simulink model "tx_chain_test"  (R2022b)
settings: Solver=FixedStepDiscrete  StartTime=0.0  StopTime=inf  RelTol=1e-3
undefined symbols (not defined in the file or in its folder): S
libraries: simrfV2elements x7, simrfV2systems x2, rfTestbenches_lib x2
settings Model: Creator=hessam  LastModifiedBy=hessam
settings DebuggingCC: InheritedTsInSrcMsg=none

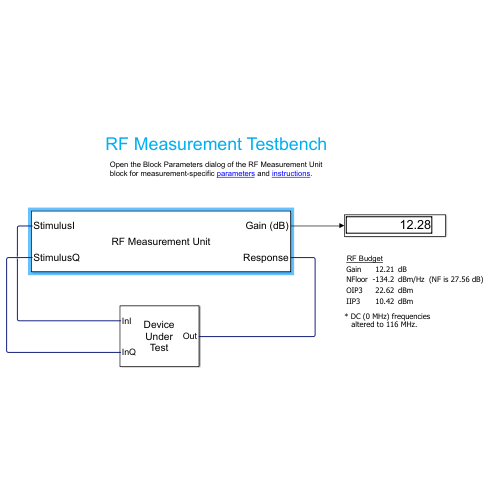
[thumbnail: Simulink's stored preview of the top-level diagram]
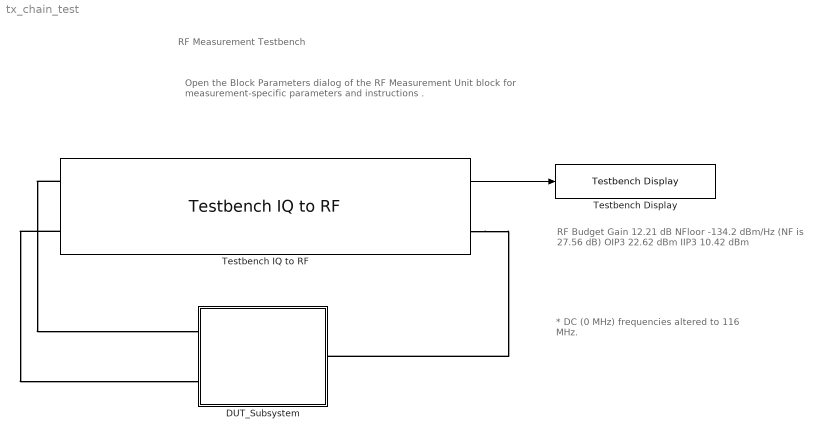
== system tx_chain_test ==
  note: RF Measurement Testbench
  note: Open the Block Parameters dialog of the RF Measurement Unit
      | block for measurement-specific parameters and instructions .
  note: * DC (0 MHz) frequencies
      | altered to 116 MHz.
  note: RF Budget
      |
      | Gain
      |
      | 12.21
      |
      | dB
      |
      | NFloor
      |
      | -134.2
      |
      | dBm/Hz
      |
      | (NF is 27.56 dB)
      |
      | OIP3
      |
      | 22.62
      |
      | dBm
      |
      | IIP3
      |
      | 10.42
      |
      | dBm
  DUT_Subsystem : Subsystem
      settings: LibrarySourceBlock=rfTestbenches_lib/simrfTestbenchIQtoRF/DUT_Subsystem
      mask Display: fprintf('Device\nUnder\nTest');
  Testbench Display : rfTestbenches_lib/simrfTestbenchIQtoRF/Testbench Display  Format=short
  Testbench IQ to RF : rfTestbenches_lib/Testbench IQ to RF  SimNoise=on  ModeStrLong=Gain  ModeStrShort=Sideband Suppression  Mode=1  IPTypeStr=Output referred  IPType=2  IQMeasureStr=I and Q (Q = -1j * I)  IQMeasure=1  InjectionTypeStr=Low-side  InjectionType=1  T_amp_dBm=0  T_amp_dBm_scL=-10  T_amp_dBm_scU=15  T_amp_dBmV=47  Fin=116e6  Fout=77e9  Base_bw=116e6  F_tone_over_Base_bw=1/8  Reset=0  ResetableRand=6.2788496288347118e-01
  wires:
  Testbench IQ to RF/1 -> Testbench Display/1
  connections:
  Testbench IQ to RF/RConn1 -- DUT_Subsystem/RConn1
  Testbench IQ to RF/LConn1 -- DUT_Subsystem/LConn1
  Testbench IQ to RF/LConn2 -- DUT_Subsystem/LConn2

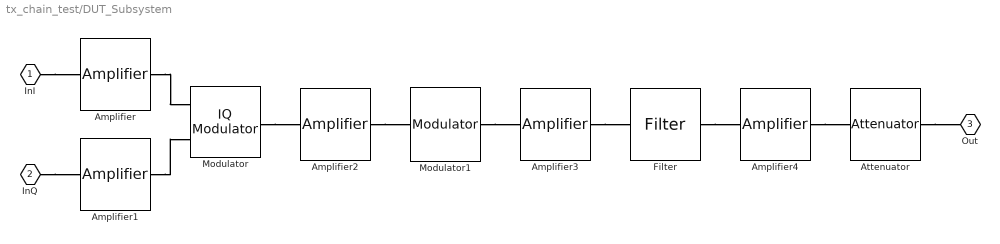
== system tx_chain_test/DUT_Subsystem ==
  Amplifier : simrfV2elements/Amplifier  classname=amplifier  DataSource=Data file  isNetworkObj=off  Paramtype=S-parameters  Sparam=[0 0;1 0]  SparamFreq=1e9 Hz  SparamZ0=50  isRationalObj=off  Residues=0  Poles=0  DF={0 0; 1 0}  Source_linear_gain=Available power gain  linear_gain=0 dB  AmAmAmPmTable=[-25,5,-1;-10,20,-2;0,27,5;5,28,12]  Zin=50  Zout=50  Source_Poly=Even and odd order  Poly_Coeffs=[0 1]  IPType=Output  IP2=Inf dBm  IP3=Inf dBm  P1dB=inf dBm  Psat=inf dBm  Gcomp=inf dBm  InternalGrounding=on  SourceFreq=Extracted from data source  PlotFreq=[1e9:1e6:3e9] Hz  PlotType=X-Y plane  YParam1=S(1,1)  YFormat1=Magnitude (dB)  YParam2=None  YFormat2=Magnitude (dB)  YOption=Linear  XOption=Linear  SparamRepresentation=Time domain (rationalfit)  FitTol=-40  FitOpt=Fit individually  MaxPoles=48  AutoImpulseLength=on  ImpulseLength=1e-10 s  MagModeling=off  AddNoise=on  NoiseType=Noise figure  NoiseDist=White  NF=25  MinNF=0  Gopt=0  RN=0  CarrierFreq=0 Hz  NoiseAutoImpulseLength=on  NoiseImpulseLength=1e-10 s  ConstS21NL=off  OpFreq=1 GHz  SetOpFreqAsMaxS21=off
  Amplifier1 : simrfV2elements/Amplifier  classname=amplifier  DataSource=Data file  isNetworkObj=off  Paramtype=S-parameters  Sparam=[0 0;1 0]  SparamFreq=1e9 Hz  SparamZ0=50  isRationalObj=off  Residues=0  Poles=0  DF={0 0; 1 0}  Source_linear_gain=Available power gain  linear_gain=0 dB  AmAmAmPmTable=[-25,5,-1;-10,20,-2;0,27,5;5,28,12]  Zin=50  Zout=50  Source_Poly=Even and odd order  Poly_Coeffs=[0 1]  IPType=Output  IP2=Inf dBm  IP3=Inf dBm  P1dB=inf dBm  Psat=inf dBm  Gcomp=inf dBm  InternalGrounding=on  SourceFreq=Extracted from data source  PlotFreq=[1e9:1e6:3e9] Hz  PlotType=X-Y plane  YParam1=S(1,1)  YFormat1=Magnitude (dB)  YParam2=None  YFormat2=Magnitude (dB)  YOption=Linear  XOption=Linear  SparamRepresentation=Time domain (rationalfit)  FitTol=-40  FitOpt=Fit individually  MaxPoles=48  AutoImpulseLength=on  ImpulseLength=1e-10 s  MagModeling=off  AddNoise=on  NoiseType=Noise figure  NoiseDist=White  NF=25  MinNF=0  Gopt=0  RN=0  CarrierFreq=0 Hz  NoiseAutoImpulseLength=on  NoiseImpulseLength=1e-10 s  ConstS21NL=off  OpFreq=1 GHz  SetOpFreqAsMaxS21=off
  Amplifier2 : simrfV2elements/Amplifier  classname=amplifier  DataSource=Data file  isNetworkObj=off  Paramtype=S-parameters  Sparam=[0 0;1 0]  SparamFreq=1e9 Hz  SparamZ0=50  isRationalObj=off  Residues=0  Poles=0  DF={0 0; 1 0}  Source_linear_gain=Available power gain  linear_gain=5 dB  AmAmAmPmTable=[-25,5,-1;-10,20,-2;0,27,5;5,28,12]  Zin=50  Zout=50  Source_Poly=Even and odd order  Poly_Coeffs=[0 1]  IPType=Output  IP2=Inf dBm  IP3=25 dBm  P1dB=inf dBm  Psat=inf dBm  Gcomp=inf dBm  InternalGrounding=on  SourceFreq=Extracted from data source  PlotFreq=[1e9:1e6:3e9] Hz  PlotType=X-Y plane  YParam1=S(1,1)  YFormat1=Magnitude (dB)  YParam2=None  YFormat2=Magnitude (dB)  YOption=Linear  XOption=Linear  SparamRepresentation=Time domain (rationalfit)  FitTol=-40  FitOpt=Fit individually  MaxPoles=48  AutoImpulseLength=on  ImpulseLength=1e-10 s  MagModeling=off  AddNoise=on  NoiseType=Noise figure  NoiseDist=White  NF=15  MinNF=0  Gopt=0  RN=0  CarrierFreq=0 Hz  NoiseAutoImpulseLength=on  NoiseImpulseLength=1e-10 s  ConstS21NL=off  OpFreq=1 GHz  SetOpFreqAsMaxS21=off
  Amplifier3 : simrfV2elements/Amplifier  classname=amplifier  DataSource=Data file  isNetworkObj=off  Paramtype=S-parameters  Sparam=[0 0;1 0]  SparamFreq=1e9 Hz  SparamZ0=50  isRationalObj=off  Residues=0  Poles=0  DF={0 0; 1 0}  Source_linear_gain=Available power gain  linear_gain=9 dB  AmAmAmPmTable=[-25,5,-1;-10,20,-2;0,27,5;5,28,12]  Zin=50  Zout=50  Source_Poly=Even and odd order  Poly_Coeffs=[0 1]  IPType=Output  IP2=Inf dBm  IP3=25 dBm  P1dB=inf dBm  Psat=inf dBm  Gcomp=inf dBm  InternalGrounding=on  SourceFreq=Extracted from data source  PlotFreq=[1e9:1e6:3e9] Hz  PlotType=X-Y plane  YParam1=S(1,1)  YFormat1=Magnitude (dB)  YParam2=None  YFormat2=Magnitude (dB)  YOption=Linear  XOption=Linear  SparamRepresentation=Time domain (rationalfit)  FitTol=-40  FitOpt=Fit individually  MaxPoles=48  AutoImpulseLength=on  ImpulseLength=1e-10 s  MagModeling=off  AddNoise=on  NoiseType=Noise figure  NoiseDist=White  NF=15  MinNF=0  Gopt=0  RN=0  CarrierFreq=0 Hz  NoiseAutoImpulseLength=on  NoiseImpulseLength=1e-10 s  ConstS21NL=off  OpFreq=1 GHz  SetOpFreqAsMaxS21=off
  Amplifier4 : simrfV2elements/Amplifier  classname=amplifier  DataSource=Data file  isNetworkObj=off  Paramtype=S-parameters  Sparam=[0 0;1 0]  SparamFreq=1e9 Hz  SparamZ0=50  isRationalObj=off  Residues=0  Poles=0  DF={0 0; 1 0}  Source_linear_gain=Available power gain  linear_gain=10 dB  AmAmAmPmTable=[-25,5,-1;-10,20,-2;0,27,5;5,28,12]  Zin=50  Zout=50  Source_Poly=Even and odd order  Poly_Coeffs=[0 1]  IPType=Output  IP2=Inf dBm  IP3=40 dBm  P1dB=inf dBm  Psat=inf dBm  Gcomp=inf dBm  InternalGrounding=on  SourceFreq=Extracted from data source  PlotFreq=[1e9:1e6:3e9] Hz  PlotType=X-Y plane  YParam1=S(1,1)  YFormat1=Magnitude (dB)  YParam2=None  YFormat2=Magnitude (dB)  YOption=Linear  XOption=Linear  SparamRepresentation=Time domain (rationalfit)  FitTol=-40  FitOpt=Fit individually  MaxPoles=48  AutoImpulseLength=on  ImpulseLength=1e-10 s  MagModeling=off  AddNoise=on  NoiseType=Noise figure  NoiseDist=White  NF=25  MinNF=0  Gopt=0  RN=0  CarrierFreq=0 Hz  NoiseAutoImpulseLength=on  NoiseImpulseLength=1e-10 s  ConstS21NL=off  OpFreq=1 GHz  SetOpFreqAsMaxS21=off
  Attenuator : simrfV2elements/Attenuator  classname=attenuator  Att=4  Zin=50  Zout=50  AddNoise=on  InternalGrounding=on
  Filter : simrfV2elements/Filter  classname=filter  DesignMethod=Butterworth  ResponseType=Bandstop  Implementation=LC Tee  ImplementationIdeal=Constant per carrier  ImplementationRational=Transfer function  UseFilterOrder=on  FilterOrder=3  PassFreq_lp=1 GHz  PassFreq_hp=2 GHz  PassFreq_bp=[2 3] GHz  PassFreq_bs=[1 4] GHz  PassAtten=10*log10(2)  StopFreq_lp=2 GHz  StopFreq_hp=1 GHz  StopFreq_bp=[1.5 3.5] GHz  StopFreq_bs=[51 55] GHz  StopAtten=40  Rsrc=100  Rload=50  AutoImpulseLength=on  ImpulseLength=1e-10 s  InternalGrounding=on  PlotFuncLeft=Voltage transfer  PlotLeftForm=Magnitude (dB)  PlotRightOnVT=None  PlotRightNoTD=None  PlotRightNoGD=None  PlotRightNoIR=None  PlotRightNoSR=None  PlotRightForm=Magnitude (dB)  FreqPoints=logspace(0,10,101)  Freq_unit=Hz  TimePoints=linspace(0,1,1e6+1)  Time_unit=s  XaxisScale=Linear  YaxisScale=Linear  needRedraw=0
  Modulator : simrfV2systems/IQ Modulator  classname=iqmod  Source_linear_gain=Available power gain  linear_gain=1 dB  Poly_Coeffs=[0 1]  LOFreq=10.884 GHz  Zin=50  Zout=50  AddIRFilters=on  AddCSFilter=on  InternalGrounding=on  ForceNextInit=off  NFloor=-149.865494556439  GainMismatch=0 dB  PhaseMismatch=0 deg  Isolation=inf dB  AddPhaseNoise=off  PhaseNoiseOffset=1  PhaseNoiseLevel=-Inf  AutoImpulseLengthPN=on  ImpulseLengthPN=1e-10  ImpulseLength_unitPN=s  Source_Poly=Even and odd order  IPType=Output  IP2=Inf dBm  IP3=15 dBm  P1dB=inf dBm  Psat=inf dBm  Gcomp=inf dBm  DesignMethodIR=Ideal  ResponseTypeIR=Lowpass  ImplementationIR=LC Tee  ImplementationIdealIR=Constant per carrier  ImplementationRationalIR=Transfer function  UseFilterOrderIR=on  FilterOrderIR=3  PassFreq_lpIR=174  PassFreq_lp_unitIR=MHz  PassFreq_hpIR=58  PassFreq_hp_unitIR=MHz  PassFreq_bpIR=[58 174]  PassFreq_bp_unitIR=MHz  PassFreq_bsIR=[21.825999999 21.942000001]  PassFreq_bs_unitIR=GHz  PassAttenIR=10*log10(2)  StopFreq_lpIR=174.000001  StopFreq_lp_unitIR=MHz  StopFreq_hpIR=57.999999  StopFreq_hp_unitIR=MHz  StopFreq_bpIR=[57.999999 174.000001]  StopFreq_bp_unitIR=MHz  StopFreq_bsIR=[21.826 21.942]  StopFreq_bs_unitIR=GHz  StopAttenIR=40  RsrcIR=50  RloadIR=50  AutoImpulseLengthIR=on  ImpulseLengthIR=1e-10  ImpulseLength_unitIR=s  DesignMethodCS=Ideal  ResponseTypeCS=Highpass  ImplementationCS=LC Tee  ImplementationIdealCS=Constant per carrier  ImplementationRationalCS=Transfer function  UseFilterOrderCS=on  FilterOrderCS=3  PassFreq_lpCS=11.058  PassFreq_lp_unitCS=GHz  PassFreq_hpCS=10.942  PassFreq_hp_unitCS=GHz  PassFreq_bpCS=[10.942 11.058]  PassFreq_bp_unitCS=GHz  PassFreq_bsCS=[10.709999999 10.826000001]  PassFreq_bs_unitCS=GHz  PassAttenCS=10*log10(2)  StopFreq_lpCS=11.058000001  StopFreq_lp_unitCS=GHz  StopFreq_hpCS=10.941999999  StopFreq_hp_unitCS=GHz  StopFreq_bpCS=[10.941999999 11.058000001]  StopFreq_bp_unitCS=GHz  StopFreq_bsCS=[10.71 10.826]  StopFreq_bs_unitCS=GHz  StopAttenCS=40  RsrcCS=50  RloadCS=50  AutoImpulseLengthCS=on  ImpulseLengthCS=1e-10  ImpulseLength_unitCS=s
  Modulator1 : simrfV2systems/Modulator  classname=rfmod  Source_linear_gain=Available power gain  linear_gain=-6 dB  Poly_Coeffs=[0 1]  LOFreq=66 GHz  Zin=50  Zout=50  AddIRFilter=on  AddCSFilter=on  InternalGrounding=on  ForceNextInit=off  Source_Poly=Even and odd order  IPType=Output  IP2=Inf dBm  IP3=15 dBm  P1dB=inf dBm  Psat=inf dBm  Gcomp=inf dBm  NF=15  Isolation=inf dB  AddPhaseNoise=off  PhaseNoiseOffset=1  PhaseNoiseLevel=-Inf  AutoImpulseLengthPN=on  ImpulseLengthPN=1e-10  ImpulseLength_unitPN=s  DesignMethodIR=Ideal  ResponseTypeIR=Lowpass  ImplementationIR=LC Tee  ImplementationIdealIR=Constant per carrier  ImplementationRationalIR=Transfer function  UseFilterOrderIR=on  FilterOrderIR=3  PassFreq_lpIR=11.058  PassFreq_lp_unitIR=GHz  PassFreq_hpIR=10.942  PassFreq_hp_unitIR=GHz  PassFreq_bpIR=[10.942 11.058]  PassFreq_bp_unitIR=GHz  PassFreq_bsIR=[142.941999999 143.058000001]  PassFreq_bs_unitIR=GHz  PassAttenIR=10*log10(2)  StopFreq_lpIR=11.058000001  StopFreq_lp_unitIR=GHz  StopFreq_hpIR=10.941999999  StopFreq_hp_unitIR=GHz  StopFreq_bpIR=[10.941999999 11.058000001]  StopFreq_bp_unitIR=GHz  StopFreq_bsIR=[142.942 143.058]  StopFreq_bs_unitIR=GHz  StopAttenIR=40  RsrcIR=50  RloadIR=50  AutoImpulseLengthIR=on  ImpulseLengthIR=1e-10  ImpulseLength_unitIR=s  DesignMethodCS=Ideal  ResponseTypeCS=Highpass  ImplementationCS=LC Tee  ImplementationIdealCS=Constant per carrier  ImplementationRationalCS=Transfer function  UseFilterOrderCS=on  FilterOrderCS=3  PassFreq_lpCS=77.058  PassFreq_lp_unitCS=GHz  PassFreq_hpCS=76.942  PassFreq_hp_unitCS=GHz  PassFreq_bpCS=[76.942 77.058]  PassFreq_bp_unitCS=GHz  PassFreq_bsCS=[54.941999999 55.058000001]  PassFreq_bs_unitCS=GHz  PassAttenCS=10*log10(2)  StopFreq_lpCS=77.058000001  StopFreq_lp_unitCS=GHz  StopFreq_hpCS=76.941999999  StopFreq_hp_unitCS=GHz  StopFreq_bpCS=[76.941999999 77.058000001]  StopFreq_bp_unitCS=GHz  StopFreq_bsCS=[54.942 55.058]  StopFreq_bs_unitCS=GHz  StopAttenCS=40  RsrcCS=50  RloadCS=50  AutoImpulseLengthCS=on  ImpulseLengthCS=1e-10  ImpulseLength_unitCS=s
  InI : PMIOPort  Side=Left
  InQ : PMIOPort  Port=2  Side=Left
  Out : PMIOPort  Port=3  Side=Right
  connections:
  InI/RConn1 -- Amplifier/LConn1
  InQ/RConn1 -- Amplifier1/LConn1
  Amplifier/RConn1 -- Modulator/LConn1
  Amplifier1/RConn1 -- Modulator/LConn2
  Modulator/RConn1 -- Amplifier2/LConn1
  Amplifier2/RConn1 -- Modulator1/LConn1
  Modulator1/RConn1 -- Amplifier3/LConn1
  Amplifier3/RConn1 -- Filter/LConn1
  Filter/RConn1 -- Amplifier4/LConn1
  Amplifier4/RConn1 -- Attenuator/LConn1
  Attenuator/RConn1 -- Out/RConn1
